simulink model "Copy_of_eCS_Algo_Simulation_2015b"  (R2015b)
settings: Solver=ode1  StartTime=0.0  StopTime=3  FixedStep=1/80000  RelTol=1e-3
PreLoadFcn:
  | if exist('tl_preloadfcn','file'), tl_preloadfcn(gcs,402); end
PostLoadFcn:
  | , if any(exist('dsrtsu_mdlpostloadfcn', 'file') == [2, 3, 6]), try dsrtsu_mdlpostloadfcn('Execute', bdroot); catch fprintf('Error in PostLoadFcn (dsrtsu_mdlpostloadfcn) for model "%s":\n %s\n', bdroot, lasterr); end, end,
  | if exist('tl_postloadfcn','file'), tl_postloadfcn(gcs,402); end
InitFcn:
  | if exist('tlds_init','file'), tlds_init(gcs); end
StartFcn:
  | if exist('tlds_start','file'), tlds_start(gcs); end
StopFcn:
  | if exist('tlds_stop','file'), tlds_stop(gcs); end
model workspace (MAT data in the model file):
  au8PrevExecProfile = [0 0 0 0 0 0]
values from neighbouring files (symbols this model uses):
  AccSensor = 5    [Parameter_eCS_Algo.m]
  AlgoType = 0    [Parameter_eCS_Algo.m]
  Cxy = 1*0.017    (= 0.017)    [Acc_Init_SelV1.m]
  Cxz = 1*0.017    (= 0.017)    [Acc_Init_SelV1.m]
  Cyx = 1*0.017    (= 0.017)    [Acc_Init_SelV1.m]
  Cyz = 1*0.017    (= 0.017)    [Acc_Init_SelV1.m]
  Czx = 1*0.017    (= 0.017)    [Acc_Init_SelV1.m]
  Czy = 1*0.017    (= 0.017)    [Acc_Init_SelV1.m]
  Forced_Oscillation = 0    [Parameter_eCS_Algo.m]    (also in run_Rotation_sim.m = run)
  FreqTemperature = 10    [Acc_Init_SelV1.m]
  MaxSensorOffset = 0.3    [Acc_Init_SelV1.m]
  Mean_x_noise = 4e-3    (= 0.004)    [Acc_Init_SelV1.m]
  Mean_y_noise = 4e-3    (= 0.004)    [Acc_Init_SelV1.m]
  Mean_z_noise = 4e-3    (= 0.004)    [Acc_Init_SelV1.m]
  ODR = 8000    [Acc_Init_SelV1.m]
  offsetcorrection_on_off = 0    [Parameter_eCS_Algo.m]
  phi_pulse_rotation = 0    [Parameter_eCS_Algo.m]    (also in run_Rotation_sim.m = angle)
  pulsetype = 2    [Parameter_eCS_Algo.m]    (also in run_simulation.m = j; run_simulation_ActiveX.m = j)
  Range = 4    [Acc_Init_SelV1.m]
  TempBias = 0    [Acc_Init_SelV1.m]
  TemperatureAmp = 0    [Acc_Init_SelV1.m]
  Var_x_noise = 1.84e-9    (= 1.84e-09)    [Acc_Init_SelV1.m]
  Var_y_noise = 2.025e-09    [Acc_Init_SelV1.m]
  Var_z_noise = 1.374e-09    [Acc_Init_SelV1.m]
  w_x = 2*pi*F_x    (= 376.991118431)    [Acc_Init_SelV1.m]
  w_y = 2*pi*F_y    (= 376.991118431)    [Acc_Init_SelV1.m]
  w_z = 2*pi*F_z    (= 376.991118431)    [Acc_Init_SelV1.m]
  x_max_temp_drift = 0.061    [Acc_Init_SelV1.m]
  x_offset_enable = 0    [Acc_Init_SelV1.m]
  x_run_to_run_drift = 0.0    (= 0)    [Acc_Init_SelV1.m]
  x_temp_co_drift = 0.000    (= 0)    [Acc_Init_SelV1.m]
  Xi_x = 0.7    [Acc_Init_SelV1.m]
  Xi_y = 0.7    [Acc_Init_SelV1.m]
  Xi_z = 0.7    [Acc_Init_SelV1.m]
  y_max_temp_drift = 0.061    [Acc_Init_SelV1.m]
  y_offset_enable = 0    [Acc_Init_SelV1.m]
  y_run_to_run_drift = 0.0    (= 0)    [Acc_Init_SelV1.m]
  y_temp_co_drift = 0.000    (= 0)    [Acc_Init_SelV1.m]
  z_max_temp_drift = 0.13    [Acc_Init_SelV1.m]
  z_offset_enable = 0    [Acc_Init_SelV1.m]
  z_run_to_run_drift = 0.0    (= 0)    [Acc_Init_SelV1.m]
  z_temp_co_drift = 0.000    (= 0)    [Acc_Init_SelV1.m]
undefined symbols (not defined in the file or in its folder): controller_sample_rate, ddv, DiscIntNeverNeededParam, ECE_L_0_x, ECE_L_0_y, ECE_L_0_z, ECE_L_45_time, ECE_L_45_x, ECE_L_45_y, ECE_L_45_z, FMVSS_45_time, FMVSS_45_x, FMVSS_45_y, FMVSS_45_z, gmw_roada_x__m_s__, gmw_roada_y__m_s__, gmw_roadtime_2kHz, KSF_50_a_x, KSF_50_a_y, KSF_50_time, KSG_30_a_x, KSG_30_a_y, KSG_30_time, Meldorf_HindenburgstraAcceleration_x__m_s_2_, Meldorf_HindenburgstraAcceleration_y__m_s_2_, Meldorf_HindenburgstraAcceleration_z__m_s_2_, Meldorf_HindenburgstraTime__s_, pulse_FF27, pulse_MPDB, pulse_ODB40, pulse_ODB64, pulse_USNCAP, pulsetime_FF27, pulsetime_MPDB, pulsetime_ODB40, pulsetime_ODB64, pulsetime_USNCAP, Rauasphalt_60_a_x, Rauasphalt_60_a_y, Rauasphalt_60_time, sigbuilder_block, TimeArray, VW_416_2kHza_x_2kHz, VW_416_2kHza_y_2kHz, VW_416_2kHztime_2kHz
libraries: simulink x40, tllib x10, tl_autosar_lib x7, simulink_extras x5, LIB_TF_G_111 x2, LIB_TF_G_12_StepControl x2, LIB_TF_G_112 x1, dspsigops x1
(part 3 of 9)

== system Copy_of_eCS_Algo_Simulation_2015b/eCS_Targetlink/Subsystem/eCS_Targetlink ==
  Ax (m.s-2) : Inport  mask(TL_Inport){data={'logdata',{'loggingmode',1},'output',{'max',39.228,'min',-39.228,'scaling','MperSecSqd_Algo/scAccel_SI'},'date',738071.59304150462}}
      settings: DeleteFcn=if exist('delete_tlblock','file')==2,delete_tlblock(gcbh);end  OpenFcn=if exist('tl_open_blockdlg','file')==2,tl_open_blockdlg(gcbh);else,open_system(gcbh,'parameter');end
      settings: CopyFcn=|
      | if exist('tl_reset_reviewflag','file')==2
      |     tl_reset_reviewflag(gcbh);
      | end
      | if exist('tl_check_ports','file')
      |     tl_check_ports(gcbh);
      | end
      settings: NameChangeFcn=|
      | if exist('rename_tlblock','file')==2,rename_tlblock(gcbh);end
      | if exist('tl_check_ports','file'), tl_check_ports(gcbh); end
      mask Help: eval(['if exist(''tl_online_help'',''file'') == 2, tl_online_help(''Topic'',''TL_Inport''),else, web([''jar:file:///'',matlabroot,''/help/toolbox/simulink/help.jar!/slref/' lower(get_param(gcbh,'Blocktype')) '.html''], ''-helpbrowser''),end'])
      mask Display: plot([0.2 0.35 NaN 0.65 0.8],[0 1 NaN 0 1]);
  Ay (m.s-2) : Inport  Port=2  mask(TL_Inport){data={'logdata',{'loggingmode',1},'output',{'max',39.228,'min',-39.228,'scaling','MperSecSqd_Algo/scAccel_SI'},'date',738071.59304170136}}
      settings: DeleteFcn=if exist('delete_tlblock','file')==2,delete_tlblock(gcbh);end  OpenFcn=if exist('tl_open_blockdlg','file')==2,tl_open_blockdlg(gcbh);else,open_system(gcbh,'parameter');end
      settings: CopyFcn=|
      | if exist('tl_reset_reviewflag','file')==2
      |     tl_reset_reviewflag(gcbh);
      | end
      | if exist('tl_check_ports','file')
      |     tl_check_ports(gcbh);
      | end
      settings: NameChangeFcn=|
      | if exist('rename_tlblock','file')==2,rename_tlblock(gcbh);end
      | if exist('tl_check_ports','file'), tl_check_ports(gcbh); end
      mask Help: eval(['if exist(''tl_online_help'',''file'') == 2, tl_online_help(''Topic'',''TL_Inport''),else, web([''jar:file:///'',matlabroot,''/help/toolbox/simulink/help.jar!/slref/' lower(get_param(gcbh,'Blocktype')) '.html''], ''-helpbrowser''),end'])
      mask Display: plot([0.2 0.35 NaN 0.65 0.8],[0 1 NaN 0 1]);
  Az (m.s-2) : Inport  Port=3  mask(TL_Inport){data={'logdata',{'loggingmode',1},'output',{'max',39.228,'min',-39.228,'scaling','MperSecSqd_Algo/scAccel_SI'},'date',738071.59304170136}}
      settings: DeleteFcn=if exist('delete_tlblock','file')==2,delete_tlblock(gcbh);end  OpenFcn=if exist('tl_open_blockdlg','file')==2,tl_open_blockdlg(gcbh);else,open_system(gcbh,'parameter');end
      settings: CopyFcn=|
      | if exist('tl_reset_reviewflag','file')==2
      |     tl_reset_reviewflag(gcbh);
      | end
      | if exist('tl_check_ports','file')
      |     tl_check_ports(gcbh);
      | end
      settings: NameChangeFcn=|
      | if exist('rename_tlblock','file')==2,rename_tlblock(gcbh);end
      | if exist('tl_check_ports','file'), tl_check_ports(gcbh); end
      mask Help: eval(['if exist(''tl_online_help'',''file'') == 2, tl_online_help(''Topic'',''TL_Inport''),else, web([''jar:file:///'',matlabroot,''/help/toolbox/simulink/help.jar!/slref/' lower(get_param(gcbh,'Blocktype')) '.html''], ''-helpbrowser''),end'])
      mask Display: plot([0.2 0.35 NaN 0.65 0.8],[0 1 NaN 0 1]);
  eCS_Algo_in_m_per_s-2 : Subsystem
  sBall : Outport  mask(TL_Outport){data={'logdata',{'loggingmode',1},'output',{'name','s16BallPosition','lsb',0.0001,'arb',1,'unit','mm'},'date',738071.5930540046}}
      settings: DeleteFcn=if exist('delete_tlblock','file')==2,delete_tlblock(gcbh);end  OpenFcn=if exist('tl_open_blockdlg','file')==2,tl_open_blockdlg(gcbh);else,open_system(gcbh,'parameter');end
      settings: CopyFcn=|
      | if exist('tl_reset_reviewflag','file')==2
      |     tl_reset_reviewflag(gcbh);
      | end
      | if exist('tl_check_ports','file')
      |     tl_check_ports(gcbh);
      | end
      settings: NameChangeFcn=|
      | if exist('rename_tlblock','file')==2,rename_tlblock(gcbh);end
      | if exist('tl_check_ports','file'), tl_check_ports(gcbh); end
      mask Help: eval(['if exist(''tl_online_help'',''file'') == 2, tl_online_help(''Topic'',''TL_Outport''),else, web([''jar:file:///'',matlabroot,''/help/toolbox/simulink/help.jar!/slref/' lower(get_param(gcbh,'Blocktype')) '.html''], ''-helpbrowser''),end'])
      mask Display: plot([0.2 0.35 NaN 0.65 0.8],[0 1 NaN 0 1]);
  b8eCSTrigg : Outport  Port=2  mask(TL_Outport){data={'logdata',{'loggingmode',1},'output',{'name','b8eCSTrigger','type','Bool','unit','mm'},'date',738072.57237952552}}
      settings: DeleteFcn=if exist('delete_tlblock','file')==2,delete_tlblock(gcbh);end  OpenFcn=if exist('tl_open_blockdlg','file')==2,tl_open_blockdlg(gcbh);else,open_system(gcbh,'parameter');end
      settings: CopyFcn=|
      | if exist('tl_reset_reviewflag','file')==2
      |     tl_reset_reviewflag(gcbh);
      | end
      | if exist('tl_check_ports','file')
      |     tl_check_ports(gcbh);
      | end
      settings: NameChangeFcn=|
      | if exist('rename_tlblock','file')==2,rename_tlblock(gcbh);end
      | if exist('tl_check_ports','file'), tl_check_ports(gcbh); end
      mask Help: eval(['if exist(''tl_online_help'',''file'') == 2, tl_online_help(''Topic'',''TL_Outport''),else, web([''jar:file:///'',matlabroot,''/help/toolbox/simulink/help.jar!/slref/' lower(get_param(gcbh,'Blocktype')) '.html''], ''-helpbrowser''),end'])
      mask Display: plot([0.2 0.35 NaN 0.65 0.8],[0 1 NaN 0 1]);
  wires:
  Ax (m.s-2)/1 -> eCS_Algo_in_m_per_s-2/1(Ax (m.s-2))
  Ay (m.s-2)/1 -> eCS_Algo_in_m_per_s-2/2(Ay (m.s-2))
  eCS_Algo_in_m_per_s-2/1(s_ball) -> sBall/1
  eCS_Algo_in_m_per_s-2/2(eCSTrigger) -> b8eCSTrigg/1  "eCSTrigger"
  Az (m.s-2)/1 -> eCS_Algo_in_m_per_s-2/3(Az (m.s-2))

== system Copy_of_eCS_Algo_Simulation_2015b/µC Signalverarbeitung und Algorithmus2/Calculate Onset >=Threshold/Calculate Onset x-Axis ==
  Acceleration [g] : Inport
  Detect Change : simulink/Logic and Bit Operations/Detect Change  vinit=0  OutDataTypeStr=boolean
  Faktor2 : SampleTimeMath  TsampMathOp=/  TsampMathImp=Offline Scaling Adjustment
  Gain : Gain  Gain=10000/100000
  Triggered Subsystem : Subsystem  TreatAsAtomicUnit=on
  delta x : Sum  Inputs=+-
  Onset [g/s] : Outport
  wires:
  Gain/1 -> Onset [g/s]/1
  Faktor2/1 -> Triggered Subsystem/1(In), Detect Change/1, delta x/1
  Detect Change/1 -> Triggered Subsystem/Trigger
  Triggered Subsystem/1(Out1) -> delta x/2
  delta x/1 -> Gain/1
  Acceleration [g]/1 -> Faktor2/1

== system Copy_of_eCS_Algo_Simulation_2015b/µC Signalverarbeitung und Algorithmus2/Calculate Onset >=Threshold/Calculate Onset y-Axis ==
  Acceleration [g] : Inport
  Detect Change : simulink/Logic and Bit Operations/Detect Change  vinit=0  OutDataTypeStr=boolean
  Faktor2 : SampleTimeMath  TsampMathOp=/  TsampMathImp=Offline Scaling Adjustment
  Gain : Gain  Gain=10000/100000
  Triggered Subsystem : Subsystem  TreatAsAtomicUnit=on
  delta x : Sum  Inputs=+-
  Onset [g/s] : Outport
  wires:
  Acceleration [g]/1 -> Faktor2/1
  delta x/1 -> Gain/1
  Triggered Subsystem/1(Out1) -> delta x/2
  Detect Change/1 -> Triggered Subsystem/Trigger
  Faktor2/1 -> Triggered Subsystem/1(In), delta x/1, Detect Change/1
  Gain/1 -> Onset [g/s]/1

== system Copy_of_eCS_Algo_Simulation_2015b/µC Signalverarbeitung und Algorithmus2/Calculate Onset >=Threshold/Calculate Onset z-Axis ==
  Acceleration [g] : Inport
  Detect Change : simulink/Logic and Bit Operations/Detect Change  vinit=0  OutDataTypeStr=boolean
  Faktor2 : SampleTimeMath  TsampMathOp=/  TsampMathImp=Offline Scaling Adjustment
  Gain : Gain  Gain=10000/100000
  Sample and Hold : dspsigops/Sample and Hold  Commented=on  trig=Rising edge  initCond=-controller_sample_rate  latchinput=on
  Triggered Subsystem : Subsystem  TreatAsAtomicUnit=on
  delta x : Sum  Inputs=+-
  Onset [g/s] : Outport
  wires:
  Gain/1 -> Onset [g/s]/1
  Faktor2/1 -> Triggered Subsystem/1(In), Detect Change/1, delta x/1
  Detect Change/1 -> Triggered Subsystem/Trigger
  Triggered Subsystem/1(Out1) -> delta x/2
  delta x/1 -> Gain/1
  Acceleration [g]/1 -> Faktor2/1

== system Copy_of_eCS_Algo_Simulation_2015b/FSM/Subsystem/FSM/FSM ==
  prrEcsAlgoFlag : Inport
  prrVehicleInputs : Inport  Port=2
  prrExecutedProfiles : Inport  Port=3
  BusSelector : BusSelector  OutputSignals=b8EcsFlag,u16BallPosition
  BusSelector1 : BusSelector  OutputSignals=u16Vx,u8BuckleState
  BusSelector2 : BusSelector  OutputSignals=u8ExecutedProfile,u8ExecutedProfileOld
  FSM_runCheckVehicleInputs : Subsystem  TreatAsAtomicUnit=on
  FSM_runMainFunction : Subsystem  TreatAsAtomicUnit=on
  PP_psrFsmProfile : tl_autosar_lib/SWC SenderPort  data={'softwarecomponent','AUTOLIV/SoftwareComponents/FSM/FSM','port','psrFsmProfile','date',738308.66468155093}  displaystring=FSM\npsrFsmProfile
  PP_psrSolenoidState : tl_autosar_lib/SWC SenderPort  data={'softwarecomponent','AUTOLIV/SoftwareComponents/FSM/FSM','port','psrSolenoidState','date',738308.6646808217}  displaystring=FSM\npsrSolenoidState
  RP_prrEcsAlgoFlag : tl_autosar_lib/SWC ReceiverPort  data={'softwarecomponent','AUTOLIV/SoftwareComponents/FSM/FSM','port','prrEcsAlgoFlag','date',738304.65103918978}  displaystring=FSM\nprrEcsAlgoFlag
  RP_prrExecutedProfiles : tl_autosar_lib/SWC ReceiverPort  data={'softwarecomponent','AUTOLIV/SoftwareComponents/FSM/FSM','port','prrExecutedProfiles','date',738314.4322294445}  displaystring=FSM\nprrExecutedProfiles
  RP_prrVehicleInputs : tl_autosar_lib/SWC ReceiverPort  data={'softwarecomponent','AUTOLIV/SoftwareComponents/FSM/FSM','port','prrVehicleInputs','date',738304.65103979164}  displaystring=FSM\nprrVehicleInputs
  psrSolenoidState : Outport
  psrFsmProfile : Outport  Port=2
  wires:
  prrEcsAlgoFlag/1 -> RP_prrEcsAlgoFlag/1
  RP_prrEcsAlgoFlag/1 -> BusSelector/1
  prrVehicleInputs/1 -> RP_prrVehicleInputs/1
  RP_prrVehicleInputs/1 -> BusSelector1/1
  BusSelector/1 -> FSM_runMainFunction/1(drparg_b8EcsFlag)  "<b8EcsFlag>"
  BusSelector1/1 -> FSM_runCheckVehicleInputs/1(drparg_u16Vx)  "<u16Vx>"
  BusSelector1/2 -> FSM_runCheckVehicleInputs/2(drparg_u8BuckleState)  "<u8BuckleState>"
  FSM_runCheckVehicleInputs/1(ab8IsSolenoidUsed) -> FSM_runMainFunction/2(ab8IsSolenoidUsed)  "ab8IsSolenoidUsed"
  PP_psrSolenoidState/1 -> psrSolenoidState/1
  PP_psrFsmProfile/1 -> psrFsmProfile/1
  FSM_runMainFunction/1(au8FsmState) -> PP_psrSolenoidState/1  "au8SolenoidState"
  FSM_runMainFunction/2(au8SelectedProfile) -> PP_psrFsmProfile/1  "au8SelectedProfile"
  prrExecutedProfiles/1 -> RP_prrExecutedProfiles/1
  RP_prrExecutedProfiles/1 -> BusSelector2/1
  BusSelector2/1 -> FSM_runMainFunction/3(drparg_u8ExecutedProfile)  "<u8ExecutedProfile>"
  BusSelector2/2 -> FSM_runMainFunction/4(drparg_u8ExecutedProfileOld)  "<u8ExecutedProfileOld>"

== system Copy_of_eCS_Algo_Simulation_2015b/SAD/Subsystem/SAD/SAD ==
  prrFsmProfile : Inport
  SAD_runMainFunction : Subsystem  TreatAsAtomicUnit=on
  psrExecutedProfiles : Outport
  wires:
  SAD_runMainFunction/1(psrExecutedProfiles) -> psrExecutedProfiles/1
  prrFsmProfile/1 -> SAD_runMainFunction/1(prrFsmProfile)

== system Copy_of_eCS_Algo_Simulation_2015b/eCS_Targetlink/Subsystem/eCS_Targetlink/eCS_Algo_in_m_per_s-2 ==
  Ax (m.s-2) : Inport  OutMin=[-39.228]  OutMax=[39.228]
  Ay (m.s-2) : Inport  Port=2
  Az (m.s-2) : Inport  Port=3
  BallAlgo : Subsystem  TreatAsAtomicUnit=on
  Constant : Constant  Value=ddv('eCS_CFG/KS16_AZ_LOCK_THRS')  mask(TL_Constant){data={'output',{'variable','eCS_CFG/KS16_AZ_LOCK_THRS'},'date',738072.37348560186}}
      settings: CopyFcn=if exist('tl_reset_reviewflag') == 2, tl_reset_reviewflag(gcbh); end  DeleteFcn=if exist('delete_tlblock','file')==2,delete_tlblock(gcbh);end  NameChangeFcn=if exist('rename_tlblock','file')==2,rename_tlblock(gcbh);end  OpenFcn=if exist('tl_open_blockdlg','file')==2,tl_open_blockdlg(gcbh);else,open_system(gcbh,'parameter');end
      mask Help: eval(['if exist(''tl_online_help'',''file'') == 2, tl_online_help(''Topic'',''TL_Constant''),else, web([''jar:file:///'',matlabroot,''/help/toolbox/simulink/help.jar!/slref/' lower(get_param(gcbh,'Blocktype')) '.html''], ''-helpbrowser''),end'])
      mask Display: plot([-0.1, 1.05, NaN, -0.1, 1.05],[.01, .01, NaN, .99, .99]);
  Crash Acceleration : Subsystem  TreatAsAtomicUnit=on
  Mux : Mux  Inputs=2
  Relational Operator : RelationalOperator  OutDataTypeStr=boolean  mask(TL_RelationalOperator){data={'date',738072.3736347917}}
      settings: DeleteFcn=if exist('delete_tlblock','file')==2,delete_tlblock(gcbh);end  NameChangeFcn=if exist('rename_tlblock','file')==2,rename_tlblock(gcbh);end  OpenFcn=if exist('tl_open_blockdlg','file')==2,tl_open_blockdlg(gcbh);else,open_system(gcbh,'parameter');end
      mask Help: eval(['if exist(''tl_online_help'',''file'') == 2, tl_online_help(''Topic'',''TL_RelationalOperator''),else, web([''jar:file:///'',matlabroot,''/help/toolbox/simulink/help.jar!/slref/' lower(get_param(gcbh,'Blocktype')) '.html''], ''-helpbrowser''),end'])
      mask Display: plot([-0.1, 1.05, NaN, -0.1, 1.05],[.01, .01, NaN, .99, .99]);
  eCS Latch Output : Subsystem  TreatAsAtomicUnit=on
  mToMm : Gain  Gain=ddv('MToMM')  mask(TL_Gain){data={'output',{'type','UInt16','lsb',2^-15,'unit','m'},'gain',{'variable','MToMM'},'date',738072.37581665511}}
      settings: CopyFcn=if exist('tl_reset_reviewflag') == 2, tl_reset_reviewflag(gcbh); end  DeleteFcn=if exist('delete_tlblock','file')==2,delete_tlblock(gcbh);end  NameChangeFcn=if exist('rename_tlblock','file')==2,rename_tlblock(gcbh);end  OpenFcn=if exist('tl_open_blockdlg','file')==2,tl_open_blockdlg(gcbh);else,open_system(gcbh,'parameter');end
      mask Help: eval(['if exist(''tl_online_help'',''file'') == 2, tl_online_help(''Topic'',''TL_Gain''),else, web([''jar:file:///'',matlabroot,''/help/toolbox/simulink/help.jar!/slref/' lower(get_param(gcbh,'Blocktype')) '.html''], ''-helpbrowser''),end'])
      mask Display: plot([0, .88, 0],[.05, .5, .93]);
  mergedTrigger : Logic  Operator=OR  AllPortsSameDT=off  OutDataTypeStr=boolean  mask(TL_LogicalOperator){data={'date',738086.66135585646}}
      settings: DeleteFcn=if exist('delete_tlblock','file')==2,delete_tlblock(gcbh);end  NameChangeFcn=if exist('rename_tlblock','file')==2,rename_tlblock(gcbh);end  OpenFcn=if exist('tl_open_blockdlg','file')==2,tl_open_blockdlg(gcbh);else,open_system(gcbh,'parameter');end
      mask Help: eval(['if exist(''tl_online_help'',''file'') == 2, tl_online_help(''Topic'',''TL_LogicalOperator''),else, web([''jar:file:///'',matlabroot,''/help/toolbox/simulink/help.jar!/slref/' lower(get_param(gcbh,'Blocktype')) '.html''], ''-helpbrowser''),end'])
      mask Display: plot([-0.1, 1.05, NaN, -0.1, 1.05],[.01, .01, NaN, .99, .99]);
  s_ball : Outport
  eCSTrigger : Outport  Port=2
  wires:
  Ax (m.s-2)/1 -> Crash Acceleration/1(Ax), Mux/1
  mToMm/1 -> s_ball/1
  Mux/1 -> BallAlgo/1(Pulses(x,y))
  Ay (m.s-2)/1 -> Crash Acceleration/2(Ay), Mux/2
  BallAlgo/1(BallPosition(m)) -> mToMm/1
  Crash Acceleration/1(b8CrashTrigger) -> mergedTrigger/2
  BallAlgo/2(BallPosTrigger) -> mergedTrigger/1
  Az (m.s-2)/1 -> Relational Operator/1
  Constant/1 -> Relational Operator/2
  Relational Operator/1 -> eCS Latch Output/2(b8IsAzLockReq)
  mergedTrigger/1 -> eCS Latch Output/1(b8eCSTrigger)
  eCS Latch Output/1(b8eCSTriggerFiltered) -> eCSTrigger/1

== system Copy_of_eCS_Algo_Simulation_2015b/µC Signalverarbeitung und Algorithmus2/Calculate Onset >=Threshold/Calculate Onset x-Axis/Triggered Subsystem ==
  In : Inport  LatchByDelayingOutsideSignal=on
  Trigger : TriggerPort
  Out1 : Outport
  wires:
  In/1 -> Out1/1

== system Copy_of_eCS_Algo_Simulation_2015b/µC Signalverarbeitung und Algorithmus2/Calculate Onset >=Threshold/Calculate Onset y-Axis/Triggered Subsystem ==
  In : Inport  LatchByDelayingOutsideSignal=on
  Trigger : TriggerPort
  Out1 : Outport
  wires:
  In/1 -> Out1/1

== system Copy_of_eCS_Algo_Simulation_2015b/µC Signalverarbeitung und Algorithmus2/Calculate Onset >=Threshold/Calculate Onset z-Axis/Triggered Subsystem ==
  In : Inport  LatchByDelayingOutsideSignal=on
  Trigger : TriggerPort
  Out1 : Outport
  wires:
  In/1 -> Out1/1

== system Copy_of_eCS_Algo_Simulation_2015b/FSM/Subsystem/FSM/FSM/FSM_runCheckVehicleInputs ==
  drparg_u16Vx : Inport  PortDimensions=1  mask(TL_Inport){data={'autosar',{'useautosarcommunication',1,'senderreceiverport','prrVehicleInputs','dataelement','u16Vx'},'date',738304.70202324074}}
      settings: CopyFcn=if exist('tl_reset_reviewflag') == 2, tl_reset_reviewflag(gcbh); end  DeleteFcn=if exist('delete_tlblock','file')==2,delete_tlblock(gcbh);end  NameChangeFcn=if exist('rename_tlblock','file')==2,rename_tlblock(gcbh);end  OpenFcn=if exist('tl_open_blockdlg','file')==2,tl_open_blockdlg(gcbh);else,open_system(gcbh,'parameter');end
      mask Help: eval(['if exist(''tl_online_help'',''file'') == 2, tl_online_help(''Topic'',''TL_Inport''),else, web([''jar:file:///'',matlabroot,''/help/toolbox/simulink/help.jar!/slref/' lower(get_param(gcbh,'Blocktype')) '.html''], ''-helpbrowser''),end'])
      mask Display: plot([0.2 0.35 NaN 0.65 0.8],[0 1 NaN 0 1]);
  drparg_u8BuckleState : Inport  Port=2  PortDimensions=1  mask(TL_Inport){data={'autosar',{'useautosarcommunication',1,'senderreceiverport','prrVehicleInputs','dataelement','u8BuckleState'},'date',738304.7020236227}}
      settings: CopyFcn=if exist('tl_reset_reviewflag') == 2, tl_reset_reviewflag(gcbh); end  DeleteFcn=if exist('delete_tlblock','file')==2,delete_tlblock(gcbh);end  NameChangeFcn=if exist('rename_tlblock','file')==2,rename_tlblock(gcbh);end  OpenFcn=if exist('tl_open_blockdlg','file')==2,tl_open_blockdlg(gcbh);else,open_system(gcbh,'parameter');end
      mask Help: eval(['if exist(''tl_online_help'',''file'') == 2, tl_online_help(''Topic'',''TL_Inport''),else, web([''jar:file:///'',matlabroot,''/help/toolbox/simulink/help.jar!/slref/' lower(get_param(gcbh,'Blocktype')) '.html''], ''-helpbrowser''),end'])
      mask Display: plot([0.2 0.35 NaN 0.65 0.8],[0 1 NaN 0 1]);
  For Iterator Subsystem : Subsystem  TreatAsAtomicUnit=on
  Runnable : tllib/Function  data={'autosar',{'useautosarspecification',1,'softwarecomponent','AUTOLIV/SoftwareComponents/FSM/FSM','runnable','FSM_runCheckVehicleInputs'},'date',738304.7020226157}  displayString=RUNNABLE
  ab8IsSolenoidUsed : Outport  PortDimensions=6  mask(TL_Outport){data={'logdata',{'loggingmode',1},'autosar',{'useautosarcommunication',1,'kind',3,'interrunnablevariable','ab8IsSolenoidUsed'},'date',738307.73139565974}}
      settings: CopyFcn=if exist('tl_reset_reviewflag') == 2, tl_reset_reviewflag(gcbh); end  DeleteFcn=if exist('delete_tlblock','file')==2,delete_tlblock(gcbh);end  NameChangeFcn=if exist('rename_tlblock','file')==2,rename_tlblock(gcbh);end  OpenFcn=if exist('tl_open_blockdlg','file')==2,tl_open_blockdlg(gcbh);else,open_system(gcbh,'parameter');end
      mask Help: eval(['if exist(''tl_online_help'',''file'') == 2, tl_online_help(''Topic'',''TL_Outport''),else, web([''jar:file:///'',matlabroot,''/help/toolbox/simulink/help.jar!/slref/' lower(get_param(gcbh,'Blocktype')) '.html''], ''-helpbrowser''),end'])
      mask Display: plot([0.2 0.35 NaN 0.65 0.8],[0 1 NaN 0 1]);
  wires:
  drparg_u16Vx/1 -> For Iterator Subsystem/1(u16Vx)
  drparg_u8BuckleState/1 -> For Iterator Subsystem/2(u8BuckleState)
  For Iterator Subsystem/1(ab8SolenoidEnable) -> ab8IsSolenoidUsed/1

== system Copy_of_eCS_Algo_Simulation_2015b/FSM/Subsystem/FSM/FSM/FSM_runMainFunction ==
  drparg_b8EcsFlag : Inport  PortDimensions=1  mask(TL_Inport){data={'autosar',{'useautosarcommunication',1,'senderreceiverport','prrEcsAlgoFlag','dataelement','b8EcsFlag'},'date',738304.65103487263}}
      settings: CopyFcn=if exist('tl_reset_reviewflag') == 2, tl_reset_reviewflag(gcbh); end  DeleteFcn=if exist('delete_tlblock','file')==2,delete_tlblock(gcbh);end  NameChangeFcn=if exist('rename_tlblock','file')==2,rename_tlblock(gcbh);end  OpenFcn=if exist('tl_open_blockdlg','file')==2,tl_open_blockdlg(gcbh);else,open_system(gcbh,'parameter');end
      mask Help: eval(['if exist(''tl_online_help'',''file'') == 2, tl_online_help(''Topic'',''TL_Inport''),else, web([''jar:file:///'',matlabroot,''/help/toolbox/simulink/help.jar!/slref/' lower(get_param(gcbh,'Blocktype')) '.html''], ''-helpbrowser''),end'])
      mask Display: plot([0.2 0.35 NaN 0.65 0.8],[0 1 NaN 0 1]);
  ab8IsSolenoidUsed : Inport  Port=2  PortDimensions=6  mask(TL_Inport){data={'autosar',{'useautosarcommunication',1,'kind',3,'interrunnablevariable','ab8IsSolenoidUsed'},'date',738307.71878736117}}
      settings: CopyFcn=if exist('tl_reset_reviewflag') == 2, tl_reset_reviewflag(gcbh); end  DeleteFcn=if exist('delete_tlblock','file')==2,delete_tlblock(gcbh);end  NameChangeFcn=if exist('rename_tlblock','file')==2,rename_tlblock(gcbh);end  OpenFcn=if exist('tl_open_blockdlg','file')==2,tl_open_blockdlg(gcbh);else,open_system(gcbh,'parameter');end
      mask Help: eval(['if exist(''tl_online_help'',''file'') == 2, tl_online_help(''Topic'',''TL_Inport''),else, web([''jar:file:///'',matlabroot,''/help/toolbox/simulink/help.jar!/slref/' lower(get_param(gcbh,'Blocktype')) '.html''], ''-helpbrowser''),end'])
      mask Display: plot([0.2 0.35 NaN 0.65 0.8],[0 1 NaN 0 1]);
  drparg_u8ExecutedProfile : Inport  Port=3  PortDimensions=6  mask(TL_Inport){data={'autosar',{'useautosarcommunication',1,'senderreceiverport','prrExecutedProfiles','dataelement','u8ExecutedProfile'},'date',738344.68576516199}}
      settings: CopyFcn=if exist('tl_reset_reviewflag') == 2, tl_reset_reviewflag(gcbh); end  DeleteFcn=if exist('delete_tlblock','file')==2,delete_tlblock(gcbh);end  NameChangeFcn=if exist('rename_tlblock','file')==2,rename_tlblock(gcbh);end  OpenFcn=if exist('tl_open_blockdlg','file')==2,tl_open_blockdlg(gcbh);else,open_system(gcbh,'parameter');end
      mask Help: eval(['if exist(''tl_online_help'',''file'') == 2, tl_online_help(''Topic'',''TL_Inport''),else, web([''jar:file:///'',matlabroot,''/help/toolbox/simulink/help.jar!/slref/' lower(get_param(gcbh,'Blocktype')) '.html''], ''-helpbrowser''),end'])
      mask Display: plot([0.2 0.35 NaN 0.65 0.8],[0 1 NaN 0 1]);
  drparg_u8ExecutedProfileOld : Inport  Port=4  PortDimensions=6  mask(TL_Inport){data={'autosar',{'useautosarcommunication',1,'senderreceiverport','prrExecutedProfiles','dataelement','u8ExecutedProfileOld'},'date',738344.68584724539}}
      settings: CopyFcn=if exist('tl_reset_reviewflag') == 2, tl_reset_reviewflag(gcbh); end  DeleteFcn=if exist('delete_tlblock','file')==2,delete_tlblock(gcbh);end  NameChangeFcn=if exist('rename_tlblock','file')==2,rename_tlblock(gcbh);end  OpenFcn=if exist('tl_open_blockdlg','file')==2,tl_open_blockdlg(gcbh);else,open_system(gcbh,'parameter');end
      mask Help: eval(['if exist(''tl_online_help'',''file'') == 2, tl_online_help(''Topic'',''TL_Inport''),else, web([''jar:file:///'',matlabroot,''/help/toolbox/simulink/help.jar!/slref/' lower(get_param(gcbh,'Blocktype')) '.html''], ''-helpbrowser''),end'])
      mask Display: plot([0.2 0.35 NaN 0.65 0.8],[0 1 NaN 0 1]);
  Determine Transition : Subsystem  TreatAsAtomicUnit=on
  ExecuteState : Subsystem  TreatAsAtomicUnit=on
  Runnable : tllib/Function  data={'autosar',{'useautosarspecification',1,'softwarecomponent','AUTOLIV/SoftwareComponents/FSM/FSM','runnable','FSM_runMainFunction'},'date',738304.65103259264}  displayString=RUNNABLE
  old state : UnitDelay  InitialCondition=ddv('FSM/astFsm/Components/au8FsmStatesOld')  SampleTime=-1  mask(TL_UnitDelay){data={'output',{'name','$D','inheritscaling',1},'state',{'variable','FSM/astFsm/Components/au8FsmStatesOld'},'date',738331.66886591434}}
      settings: CopyFcn=if exist('tl_reset_reviewflag') == 2, tl_reset_reviewflag(gcbh); end  DeleteFcn=if exist('delete_tlblock','file')==2,delete_tlblock(gcbh);end  NameChangeFcn=if exist('rename_tlblock','file')==2,rename_tlblock(gcbh);end  OpenFcn=if exist('tl_open_blockdlg','file')==2,tl_open_blockdlg(gcbh);else,open_system(gcbh,'parameter');end
      mask Help: eval(['if exist(''tl_online_help'',''file'') == 2, tl_online_help(''Topic'',''TL_UnitDelay''),else, web([''jar:file:///'',matlabroot,''/help/toolbox/simulink/help.jar!/slref/' lower(get_param(gcbh,'Blocktype')) '.html''], ''-helpbrowser''),end'])
      mask Display: plot([-0.1, 1.05, NaN, -0.1, 1.05],[.01, .01, NaN, .99, .99]);
  au8FsmState : Outport  PortDimensions=6  mask(TL_Outport){data={'logdata',{'loggingmode',1},'autosar',{'useautosarcommunication',1,'senderreceiverport','psrSolenoidState','dataelement','au8SolenoidState'},'date',738314.63122943288}}
      settings: CopyFcn=if exist('tl_reset_reviewflag') == 2, tl_reset_reviewflag(gcbh); end  DeleteFcn=if exist('delete_tlblock','file')==2,delete_tlblock(gcbh);end  NameChangeFcn=if exist('rename_tlblock','file')==2,rename_tlblock(gcbh);end  OpenFcn=if exist('tl_open_blockdlg','file')==2,tl_open_blockdlg(gcbh);else,open_system(gcbh,'parameter');end
      mask Help: eval(['if exist(''tl_online_help'',''file'') == 2, tl_online_help(''Topic'',''TL_Outport''),else, web([''jar:file:///'',matlabroot,''/help/toolbox/simulink/help.jar!/slref/' lower(get_param(gcbh,'Blocktype')) '.html''], ''-helpbrowser''),end'])
      mask Display: plot([0.2 0.35 NaN 0.65 0.8],[0 1 NaN 0 1]);
  au8SelectedProfile : Outport  Port=2  PortDimensions=6  mask(TL_Outport){data={'logdata',{'loggingmode',1},'autosar',{'useautosarcommunication',1,'senderreceiverport','psrFsmProfile','dataelement','au8SelectedProfile'},'date',738314.63131238427}}
      settings: CopyFcn=if exist('tl_reset_reviewflag') == 2, tl_reset_reviewflag(gcbh); end  DeleteFcn=if exist('delete_tlblock','file')==2,delete_tlblock(gcbh);end  NameChangeFcn=if exist('rename_tlblock','file')==2,rename_tlblock(gcbh);end  OpenFcn=if exist('tl_open_blockdlg','file')==2,tl_open_blockdlg(gcbh);else,open_system(gcbh,'parameter');end
      mask Help: eval(['if exist(''tl_online_help'',''file'') == 2, tl_online_help(''Topic'',''TL_Outport''),else, web([''jar:file:///'',matlabroot,''/help/toolbox/simulink/help.jar!/slref/' lower(get_param(gcbh,'Blocktype')) '.html''], ''-helpbrowser''),end'])
      mask Display: plot([0.2 0.35 NaN 0.65 0.8],[0 1 NaN 0 1]);
  wires:
  drparg_b8EcsFlag/1 -> Determine Transition/1(b8EcsFlag)
  ab8IsSolenoidUsed/1 -> Determine Transition/2(ab8IsSolenoidUsed)
  Determine Transition/1(au8State) -> old state/1, au8FsmState/1, ExecuteState/1(au8States)
  drparg_u8ExecutedProfile/1 -> Determine Transition/3(au8ExecutedProfiles)
  drparg_u8ExecutedProfileOld/1 -> Determine Transition/4(au8ExecutedProfilesOld)
  ExecuteState/1(au8FsmProfiles) -> au8SelectedProfile/1
  old state/1 -> Determine Transition/5(au8OldState)

== system Copy_of_eCS_Algo_Simulation_2015b/SAD/Subsystem/SAD/SAD/SAD_runMainFunction ==
  prrFsmProfile : Inport
  BusCreator : BusCreator  Inputs=2
  Demux4 : Demux  Outputs=2
  FcnCallGenerator : simulink/Ports & Subsystems/Function-Call Generator  sample_time=0.001  numberOfIterations=1
  PP_psrExecutedProfiles : tl_autosar_lib/SWC SenderPort  data={'softwarecomponent','AUTOLIV/SoftwareComponents/SAD/SAD','port','psrExecutedProfiles','date',738329.69196237263}  displaystring=SAD\npsrExecutedProfiles
  RP_prrFsmProfile : tl_autosar_lib/SWC ReceiverPort  data={'softwarecomponent','AUTOLIV/SoftwareComponents/SAD/SAD','port','prrFsmProfile','date',738331.38162996527}  displaystring=SAD\nprrFsmProfile
  SAD_runExecuteStep : Subsystem  TreatAsAtomicUnit=on
  SAD_runExtractProfileAndStep : Subsystem  TreatAsAtomicUnit=on
  Triggered Subsystem : Subsystem  TreatAsAtomicUnit=on
  psrExecutedProfiles : Outport
  wires:
  PP_psrExecutedProfiles/1 -> psrExecutedProfiles/1
  BusCreator/1 -> PP_psrExecutedProfiles/1
  prrFsmProfile/1 -> RP_prrFsmProfile/1
  SAD_runExtractProfileAndStep/3(as16SlopeValues) -> SAD_runExecuteStep/1(as16SlopeValues)  "as16SlopeValues"
  SAD_runExtractProfileAndStep/4(au16FirstOrderValues) -> SAD_runExecuteStep/2(au16FirstOrderValues)  "au16FirstOrderValues"
  SAD_runExtractProfileAndStep/5(au8OrderType) -> SAD_runExecuteStep/3(au8OrderType)  "au8OrderType"
  RP_prrFsmProfile/1 -> SAD_runExtractProfileAndStep/1(drparg_au8SelectedProfile)  "au8SelectedProfile"
  Triggered Subsystem/1(5ms) -> SAD_runExtractProfileAndStep/Trigger
  FcnCallGenerator/1 -> Demux4/1
  Demux4/1 -> SAD_runExecuteStep/Trigger
  Demux4/2 -> Triggered Subsystem/Trigger
  SAD_runExtractProfileAndStep/2(dsp_u8ExecutedProfileOld) -> BusCreator/2  "u8ExecutedProfileOld"
  SAD_runExtractProfileAndStep/1(dsp_u8ExecutedProfile) -> BusCreator/1  "u8ExecutedProfile"
  SAD_runExecuteStep/1(PrevDuty) -> SAD_runExtractProfileAndStep/2(InPort)
